simulink model "TestingModel"  (R2021a)
settings: Solver=VariableStepAuto  StartTime=0.0  StopTime=inf  RelTol=1e-3
values from neighbouring files (symbols this model uses):
  bitRate = 100e6    (= 100000000)    [PrepareLink.m]
  G_ant_rx = 40    [PrepareLink.m]
  G_ant_tx = 30    [PrepareLink.m]
undefined symbols (not defined in the file or in its folder): doppler, FSPL_TX
libraries: commfilt2 x3, commdigbbndpm3 x2, commrfcorlib x1, commrandsrc3 x1, commsink2 x1, commutil2 x1, commrflib2 x1, commchan3 x1
settings Model: Creator=drewd  LastModifiedBy=drewd

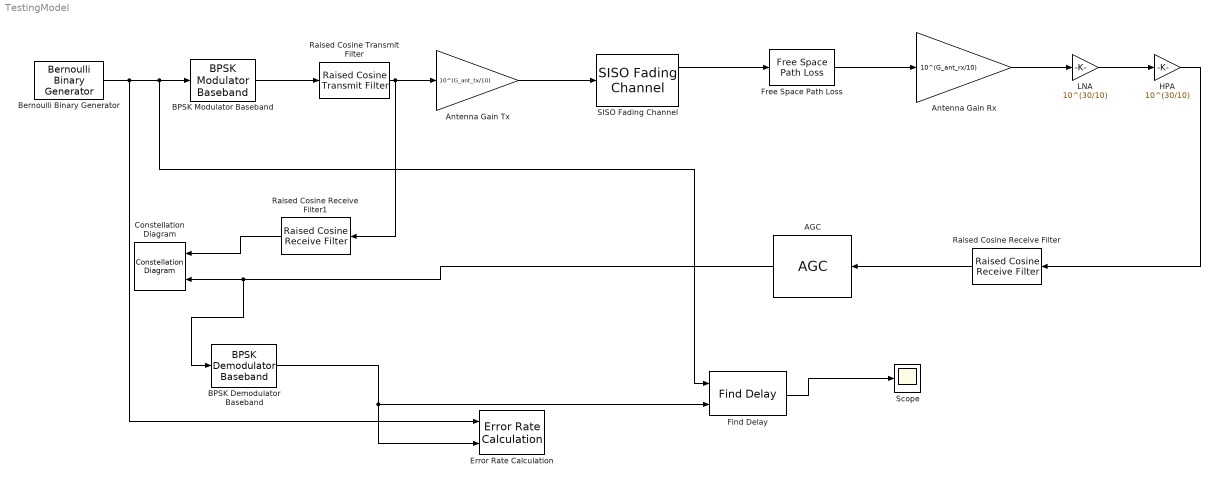
== system TestingModel ==
  AGC : commrfcorlib/AGC  LegacyMode=off  DetectorMethod=Rectifier  LoopMethod=Linear  UpdatePeriod=100  StepSize=0.1  AdaptationStepSize=0.01  DesiredOutputPower=1  AveragingLength=256  MaximumGain=30  MaxPowerGain=60  GainOutputPort=off  InputPowerOutputPort=off  SimulateUsing=Interpreted execution
  Antenna Gain Rx : Gain  Gain=10^(G_ant_rx/10)
  Antenna Gain Tx : Gain  Gain=10^(G_ant_tx/10)
  BPSK Demodulator Baseband : commdigbbndpm3/BPSK Demodulator Baseband  DecType=Hard decision  VarSource=Dialog  Variance=1  Ph=pi/2  outDtype=Inherit via internal rule  derotateFactorWordLen=16  derotateFactorDataTypeStr=Inherit: Same word length as input  derotateFactorLastDataTypeStr=Inherit: Same word length as input
  BPSK Modulator Baseband : commdigbbndpm3/BPSK Modulator Baseband  Ph=pi/2  outDtype=double  outWordLen=16  outUDDataType=sfix(16)  outFracLenMode=Best precision  outFracLen=15  outDataTypeStr=double  outLastDataTypeStr=double
  Bernoulli Binary Generator : commrandsrc3/Bernoulli Binary Generator  ProbabilityOfZero=0.5  SeedSource=Auto  Seed=0  SampleTime=1/bitRate  SamplesPerFrame=bitsPerFrame  OutputDataType=double  SimulateUsing=Interpreted execution
  Constellation Diagram : ConstellationDiagram  NumInputPorts=2
  Error Rate Calculation : commsink2/Error Rate Calculation  N=106  st_delay=0  cp_mode=Entire frame  subframe=[]  PMode=Port  WsName=ErrorVec  RsMode2=off  stop=off  numErr=100  maxBits=1e6
  Find Delay : commutil2/Find Delay  corrLength=300  chgSigOP=off  stopUpdate=off  numConstDelay=3
      settings: SourceProductBaseCode=CM
  Free Space Path Loss : commrflib2/Free Space Path Loss  mode=Distance and Frequency  dB=-FSPL_TX  d=R  fc=fc_tx
      settings: SourceProductBaseCode=CM
  HPA : Gain  Gain=10^(30/10)
  LNA : Gain  Gain=10^(30/10)
  Raised Cosine Receive Filter : commfilt2/Raised Cosine Receive Filter  filtType=Square root  R=0.2  filtSpan=6  N=8  downFactor=8  downOffset=0  filterGain=1/sqrt(8)  InputProcessing=Columns as channels (frame based)  RateOptions=Enforce single-rate processing  framing=Mute  checkCoeff=off  variableName=rcRxFilt  currentFiltSpan=10  D=5  inputOffset=0  sampMode=Mute  saveAsFlag=0  rateMode=Downsampling  checkGain=Normalized  launchFVT=on  roundingMode=Floor  overflowMode=off  coeffDataTypeStr=Inherit: Same word length as input  coeffMin=[]  coeffMax=[]  coeffLastDataTypeStr=Inherit: Same word length as input  accumDataTypeStr=Inherit: Same as product output  accumLastDataTypeStr=Inherit: Same as product output  outputDataTypeStr=Inherit: Same as accumulator  outputMin=[]  outputMax=[]  outputLastDataTypeStr=Inherit: Same as accumulator
  Raised Cosine Receive Filter1 : commfilt2/Raised Cosine Receive Filter  filtType=Square root  R=0.2  filtSpan=6  N=8  downFactor=8  downOffset=0  filterGain=1  InputProcessing=Columns as channels (frame based)  RateOptions=Enforce single-rate processing  framing=Mute  checkCoeff=off  variableName=rcRxFilt1  currentFiltSpan=10  D=5  inputOffset=0  sampMode=Mute  saveAsFlag=0  rateMode=Downsampling  checkGain=Normalized  launchFVT=on  roundingMode=Floor  overflowMode=off  coeffDataTypeStr=Inherit: Same word length as input  coeffMin=[]  coeffMax=[]  coeffLastDataTypeStr=Inherit: Same word length as input  accumDataTypeStr=Inherit: Same as product output  accumLastDataTypeStr=Inherit: Same as product output  outputDataTypeStr=Inherit: Same as accumulator  outputMin=[]  outputMax=[]  outputLastDataTypeStr=Inherit: Same as accumulator
  Raised Cosine Transmit Filter : commfilt2/Raised Cosine Transmit Filter  filtType=Square root  R=0.2  filtSpan=6  N=8  filterGain=1  InputProcessing=Columns as channels (frame based)  RateOptions=Enforce single-rate processing  framing=Mute  checkCoeff=off  variableName=rcTxFilt  checkGain=Normalized  sampMode=Mute  saveAsFlag=0  currentFiltSpan=10  D=(10)/2  launchFVT=on  roundingMode=Floor  overflowMode=off  coeffDataTypeStr=Inherit: Same word length as input  coeffMin=[]  coeffMax=[]  coeffLastDataTypeStr=Inherit: Same word length as input  outputDataTypeStr=Inherit: Same as accumulator  outputMin=[]  outputMax=[]  outputLastDataTypeStr=Inherit: Same as accumulator
  SISO Fading Channel : commchan3/SISO Fading Channel  InheritSampleRate=on  SampleRate=1  PathDelays=1e-6  AveragePathGains=-3  NormalizePathGains=on  FadingDistribution=Rician  KFactor=Kfactor  DirectPathDopplerShift=0  DirectPathInitialPhase=0  MaximumDopplerShift=0  DopplerSpectrum=doppler('Jakes')  RandomStream=mt19937ar with seed  Seed=73  PathGainsOutputPort=on  ChannelFilterDelayOutputPort=off  SimulateUsing=Interpreted execution  Visualization=Off  PathsForDopplerDisplay=1  SamplesToDisplay=25%
  Scope : Scope
  wires:
  Bernoulli Binary Generator/1 -> Error Rate Calculation/1, BPSK Modulator Baseband/1, Find Delay/1
  Free Space Path Loss/1 -> Antenna Gain Rx/1
  Antenna Gain Rx/1 -> LNA/1
  LNA/1 -> HPA/1
  BPSK Modulator Baseband/1 -> Raised Cosine Transmit Filter/1
  Raised Cosine Transmit Filter/1 -> Raised Cosine Receive Filter1/1, Antenna Gain Tx/1
  HPA/1 -> Raised Cosine Receive Filter/1
  Raised Cosine Receive Filter/1 -> AGC/1
  Antenna Gain Tx/1 -> SISO Fading Channel/1
  SISO Fading Channel/1 -> Free Space Path Loss/1
  Raised Cosine Receive Filter1/1 -> Constellation Diagram/1
  BPSK Demodulator Baseband/1 -> Find Delay/2, Error Rate Calculation/2
  Find Delay/1 -> Scope/1
  AGC/1 -> BPSK Demodulator Baseband/1, Constellation Diagram/2
